simulink model "InvertedPendulumLQR"  (R2023b)
settings: Solver=FixedStepAuto  StartTime=0.0  StopTime=inf  RelTol=1e-3
undefined symbols (not defined in the file or in its folder): LF
libraries: instrumentseriallib x3, simulink x2
settings Model: ExtModeTrigDuration=2  Creator=mattp  LastModifiedBy=mattp
settings OptimizationCC: EnhancedBackFolding=on  PassReuseOutputArgsAs=Individual arguments  ZeroExternalMemoryAtStartup=off  ZeroInternalMemoryAtStartup=off  MaxStackSize=64  OptimizeBlockOrder=speed  DifferentSizesBufferReuse=on  OptimizationCustomize=off  EfficientTunableParamExpr=on
settings DebuggingCC: ParameterPrecisionLossMsg=none  ParameterTunabilityLossMsg=error
settings HardwareCC: ProdBitPerInt=16  ProdBitPerPointer=16  ProdBitPerSizeT=16  ProdBitPerPtrDiffT=16  ProdLargestAtomicFloat=None  ProdWordSize=8  ProdHWDeviceType=Atmel->AVR  UseEmbeddedCoderFeatures=off  UseSimulinkCoderFeatures=off
settings SFSimCC: MATLABDynamicMemAlloc=off
settings RTWCC: Description=Embedded Coder  SystemTargetFile=ert.tlc  HardwareBoard=Arduino Uno  TemplateMakefile=ert_default_tmf  Toolchain=Arduino AVR
settings CodeAppCC: ForceParamTrailComments=on  IgnoreCustomStorageClasses=off  OperatorAnnotations=on  SimulinkDataObjDesc=on  SFDataObjDesc=on  InsertBlockDesc=on
settings ERTTargetCC: SupportContinuousTime=on  SupportNonInlinedSFcns=on  SupportVariableSizeSignals=on  ExtModeTransport=3  ExtModeStaticAlloc=on  ExtModeAutomaticAllocSize=off  ExtModeStaticAllocSize=250  ExtModeMexFile=ext_xcp  ExtModeIntrfLevel=Level2 - Open

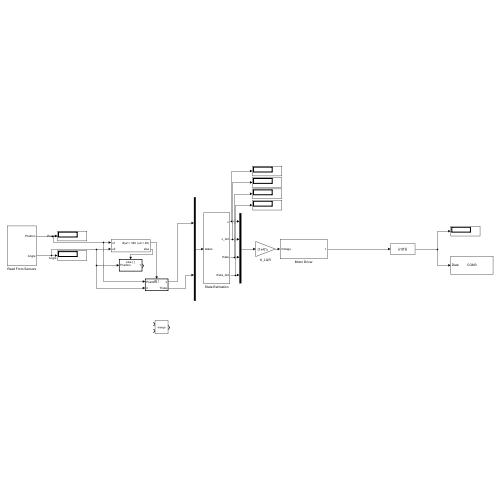
[thumbnail: Simulink's stored preview of the top-level diagram]
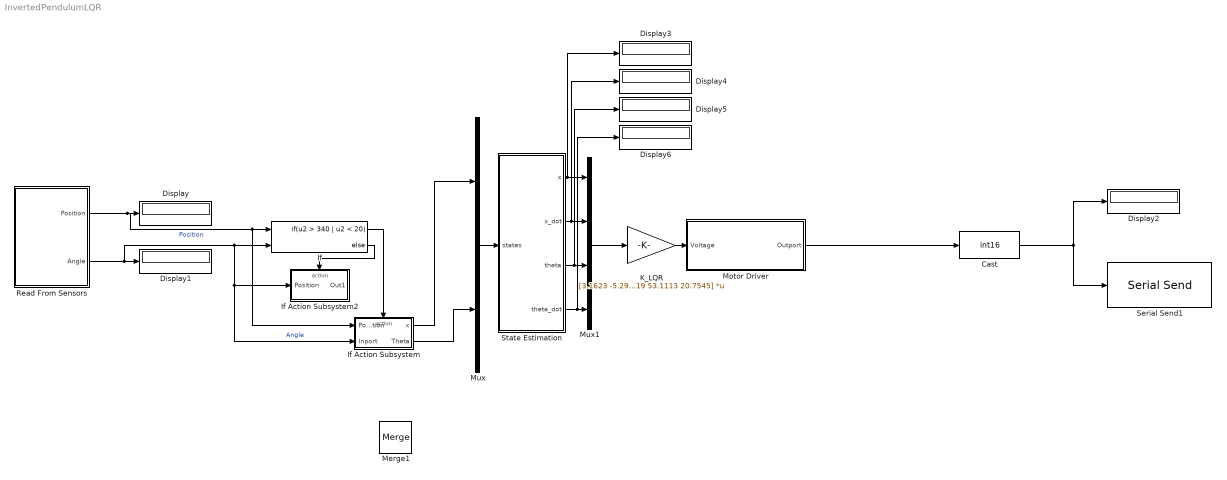
== system InvertedPendulumLQR ==
  Cast : DataTypeConversion  OutDataTypeStr=int16  SaturateOnIntegerOverflow=off  RndMeth=Floor
  Display{,1..6} (7 alike) : Display
  If : If  NumInputs=2  IfExpression=u2 > 340 | u2 < 20
  If Action Subsystem : Subsystem  TreatAsAtomicUnit=on
  If Action Subsystem2 : Subsystem  TreatAsAtomicUnit=on
  K_LQR : Gain  Gain=[3.1623 -5.2919 53.1113 20.7545]  Multiplication=Matrix(K*u)
  Merge1 : Merge
  Motor Driver : Subsystem
  Mux : Mux  Inputs=2
  Mux1 : Mux
  Read From Sensors : Subsystem
  Serial Send1 : instrumentseriallib/Serial Send  Priority=1  PortSel=COM3  Port=COM3  ComPort=COM3  Header=[]  Terminator=LF ('\n')  CustomTerminator=[]  EnableBlockingMode=on  SimulateUsing=Interpreted execution  BlockInModel=on  aMode=1
  State Estimation : Subsystem
  wires:
  Read From Sensors/1(Position) -> If/1, If Action Subsystem/1(Position), Display/1  "Position"
  Read From Sensors/2(Angle) -> If Action Subsystem2/1(Position), If Action Subsystem/2(Inport), If/2, Display1/1  "Angle"
  State Estimation/1(x) -> Display3/1, Mux1/1
  State Estimation/2(x_dot) -> Display4/1, Mux1/2
  State Estimation/3(theta) -> Display5/1, Mux1/3
  State Estimation/4(theta_dot) -> Display6/1, Mux1/4
  Mux1/1 -> K_LQR/1
  K_LQR/1 -> Motor Driver/1(Voltage)
  Mux/1 -> State Estimation/1(states)
  If/2 -> If Action Subsystem2/Action
  If Action Subsystem/1(x) -> Mux/1
  If Action Subsystem/2(Theta) -> Mux/2
  Motor Driver/1(Outport) -> Cast/1
  Cast/1 -> Serial Send1/1, Display2/1
  If/1 -> If Action Subsystem/Action

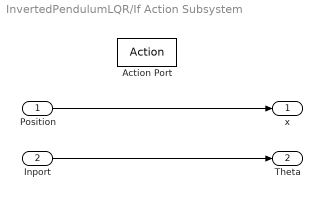
== system InvertedPendulumLQR/If Action Subsystem ==
  Position : Inport
  Inport : Inport  Port=2
  Action Port : ActionPort  ActionPortLabel=if(u2 > 340 | u2 < 20)
  x : Outport
  Theta : Outport  Port=2
  wires:
  Position/1 -> x/1
  Inport/1 -> Theta/1

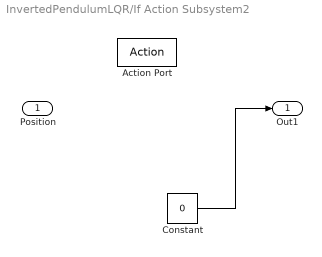
== system InvertedPendulumLQR/If Action Subsystem2 ==
  Position : Inport
  Action Port : ActionPort  ActionPortLabel=else
  Constant : Constant  Value=0  OutDataTypeStr=int16
  Out1 : Outport
  wires:
  Constant/1 -> Out1/1

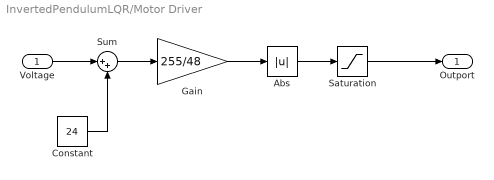
== system InvertedPendulumLQR/Motor Driver ==
  Voltage : Inport
  Abs : Abs  SaturateOnIntegerOverflow=off
  Constant : Constant  Value=24
  Gain : Gain  Gain=255/48  OutDataTypeStr=int16
  Saturation : Saturate  UpperLimit=255  LowerLimit=0
  Sum : Sum  Inputs=|++
  Outport : Outport
  wires:
  Voltage/1 -> Sum/1
  Gain/1 -> Abs/1
  Sum/1 -> Gain/1
  Constant/1 -> Sum/2
  Abs/1 -> Saturation/1
  Saturation/1 -> Outport/1

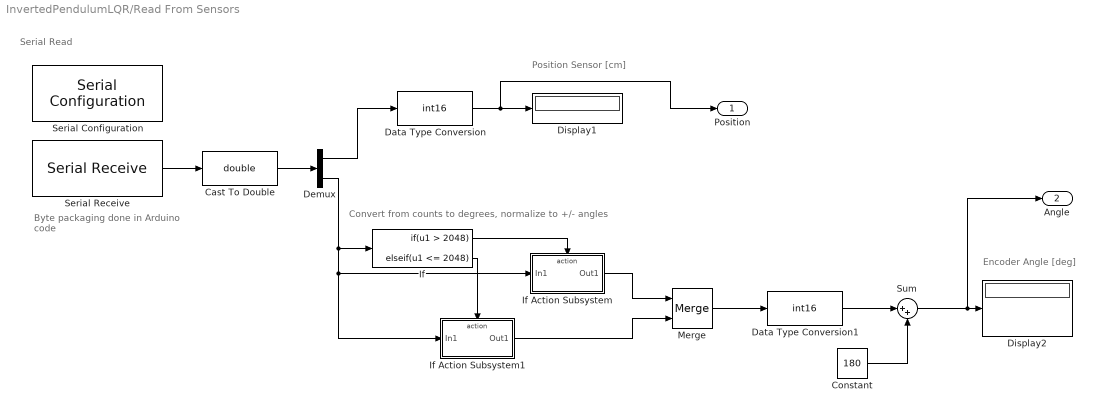
== system InvertedPendulumLQR/Read From Sensors ==
  note: Serial Read
  note: Convert from counts to degrees, normalize to +/- angles
  note: Encoder Angle [deg]
  note: Position Sensor [cm]
  note: Byte packaging done in Arduino code
  Cast To Double : DataTypeConversion  OutDataTypeStr=double  SaturateOnIntegerOverflow=off  RndMeth=Floor
  Constant : Constant  Value=180  OutDataTypeStr=int16
  Data Type Conversion : DataTypeConversion  OutDataTypeStr=int16  SaturateOnIntegerOverflow=off  RndMeth=Floor
  Data Type Conversion1 : DataTypeConversion  OutDataTypeStr=int16  SaturateOnIntegerOverflow=off  RndMeth=Floor
  Demux : Demux  Outputs=2
  Display1 : Display
  Display2 : Display
  If : If  IfExpression=u1 > 2048  ElseIfExpressions=u1 <= 2048  ShowElse=off
  If Action Subsystem : Subsystem  TreatAsAtomicUnit=on
  If Action Subsystem1 : Subsystem  TreatAsAtomicUnit=on
  Merge : Merge
  Serial Configuration : instrumentseriallib/Serial Configuration  Priority=-200000  PortSel=COM3  Port=COM3  ComPort=COM3  BaudRate=115200  DataBits=8  Parity=none  StopBits=1  ByteOrder=little-endian  FlowControl=none  Timeout=10  SimulateUsing=Interpreted execution  BlockInModel=on  aMode=1
  Serial Receive : instrumentseriallib/Serial Receive  Priority=1  PortSel=COM3  Port=COM3  ComPort=COM3  DataType=single  SaveDataType=uint8  ToggleHeader=on  Header='A'  ToggleTerminator=on  Terminator=LF ('\n')  CustomTerminator=[]  InputFormat=Column major  ToggleDataSize=on  DataSize=[1 2]  EnableBlockingMode=on  ActionDataUnavailable=Output last received value  ActionWhenDataUnavailable=Output last received value  CustomValue=0  SampleTime=0.05  SimulateUsing=Interpreted execution  BlockInModel=on  aMode=1
  Sum : Sum  Inputs=|++
  Position : Outport
  Angle : Outport  Port=2
  wires:
  Merge/1 -> Data Type Conversion1/1
  If/2 -> If Action Subsystem1/Action
  If/1 -> If Action Subsystem/Action
  Demux/2 -> If Action Subsystem1/1(In1), If Action Subsystem/1(In1), If/1
  Demux/1 -> Data Type Conversion/1
  Serial Receive/1 -> Cast To Double/1
  Data Type Conversion/1 -> Position/1, Display1/1
  Cast To Double/1 -> Demux/1
  If Action Subsystem/1(Out1) -> Merge/1
  If Action Subsystem1/1(Out1) -> Merge/2
  Data Type Conversion1/1 -> Sum/1
  Sum/1 -> Angle/1, Display2/1
  Constant/1 -> Sum/2

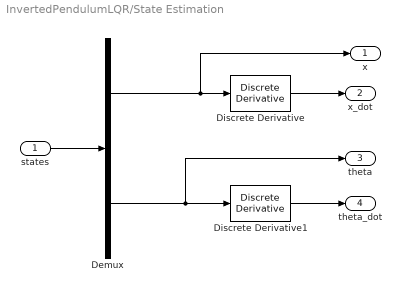
== system InvertedPendulumLQR/State Estimation ==
  states : Inport
  Demux : Demux  Outputs=2
  Discrete Derivative : simulink/Discrete/Discrete Derivative  gainval=1.0  ICPrevScaledInput=0.0  OutMin=[]  OutMax=[]  OutDataTypeStr=int16  OutputDataTypeScalingMode=int16  OutDataType=fixdt(1, 16)  OutScaling=2^-10  DoSatur=off
  Discrete Derivative1 : simulink/Discrete/Discrete Derivative  gainval=1.0  ICPrevScaledInput=0.0  OutMin=[]  OutMax=[]  OutDataTypeStr=int16  OutputDataTypeScalingMode=int16  OutDataType=fixdt(1, 16)  OutScaling=2^-10  DoSatur=off
  x : Outport
  x_dot : Outport  Port=2
  theta : Outport  Port=3
  theta_dot : Outport  Port=4
  wires:
  Discrete Derivative/1 -> x_dot/1
  Discrete Derivative1/1 -> theta_dot/1
  Demux/1 -> x/1, Discrete Derivative/1
  Demux/2 -> theta/1, Discrete Derivative1/1
  states/1 -> Demux/1

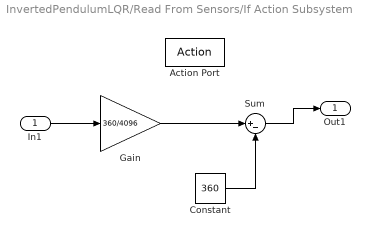
== system InvertedPendulumLQR/Read From Sensors/If Action Subsystem ==
  In1 : Inport
  Action Port : ActionPort  ActionPortLabel=if(u1 > 2048)
  Constant : Constant  Value=360
  Gain : Gain  Gain=360/4096
  Sum : Sum  Inputs=|+-
  Out1 : Outport
  wires:
  In1/1 -> Gain/1
  Gain/1 -> Sum/1
  Sum/1 -> Out1/1
  Constant/1 -> Sum/2

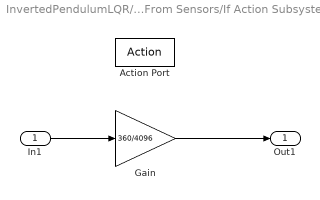
== system InvertedPendulumLQR/Read From Sensors/If Action Subsystem1 ==
  In1 : Inport
  Action Port : ActionPort  ActionPortLabel=elseif(u1 <= 2048)
  Gain : Gain  Gain=360/4096
  Out1 : Outport
  wires:
  In1/1 -> Gain/1
  Gain/1 -> Out1/1
